simulink model "mod5_counter"  (R2020b)
settings: Solver=VariableStepAuto  StartTime=0.0  StopTime=10.0  RelTol=1e-3
settings Model: Creator=ADMIN  LastModifiedBy=ADMIN

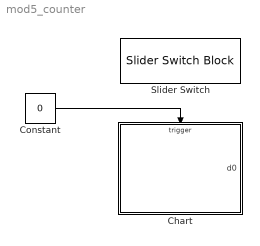
== system mod5_counter ==
  Chart : Stateflow chart  TreatAsAtomicUnit=on
  Constant : Constant  Value=0
  Slider Switch : SliderSwitchBlock
      settings: Values={{'Off', 'On'}, [0 1]}
  wires:
  Constant/1 -> Chart/Trigger

== stateflow chart mod5_counter/Chart ==
  state digit1 [parallel]
    settings: executionOrder=1
    state Zero
      en:
      d0=0;
    state One
      en:
      d0=1;
    state Two
      en:
      d0=2;
    state Four
      d0=4;
    state Three
      en:
      d0=3;
    (default) -> Zero
    Zero -> One : InputClick
    One -> Two : InputClick
    Four -> Zero : InputClick
    Two -> Three : InputClick
    Three -> Four : InputClick
  state digit2 [parallel]
    settings: executionOrder=2
  state digit3 [parallel]
    settings: executionOrder=3
  data: d0 output
  events: InputClick input FUNCTION_CALL_EVENT
